simulink subsystem "Modulador_Tensiones"  (R2026a)
settings: Solver=VariableStepAuto
values from neighbouring files (symbols this model uses):
  L_d = 6.6e-3    (= 0.0066)    [coeficientes.m]
  L_q = 5.8e-3    (= 0.0058)    [coeficientes.m]
  lambda = 0.016    [coeficientes.m]
  Pp = 3    [coeficientes.m]
libraries: eeTransforms x2
settings Model: Creator=admin  LastModifiedBy=admin

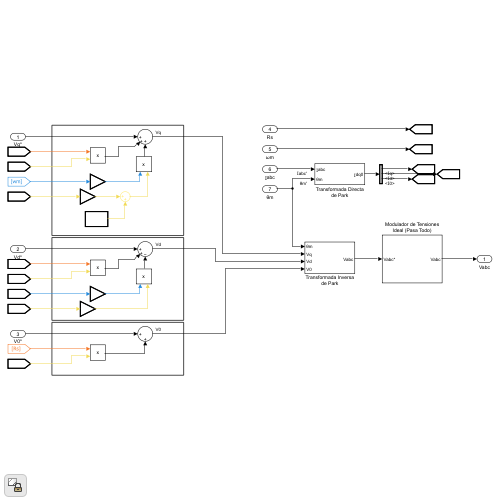
[thumbnail: Simulink's stored preview of the top-level diagram]
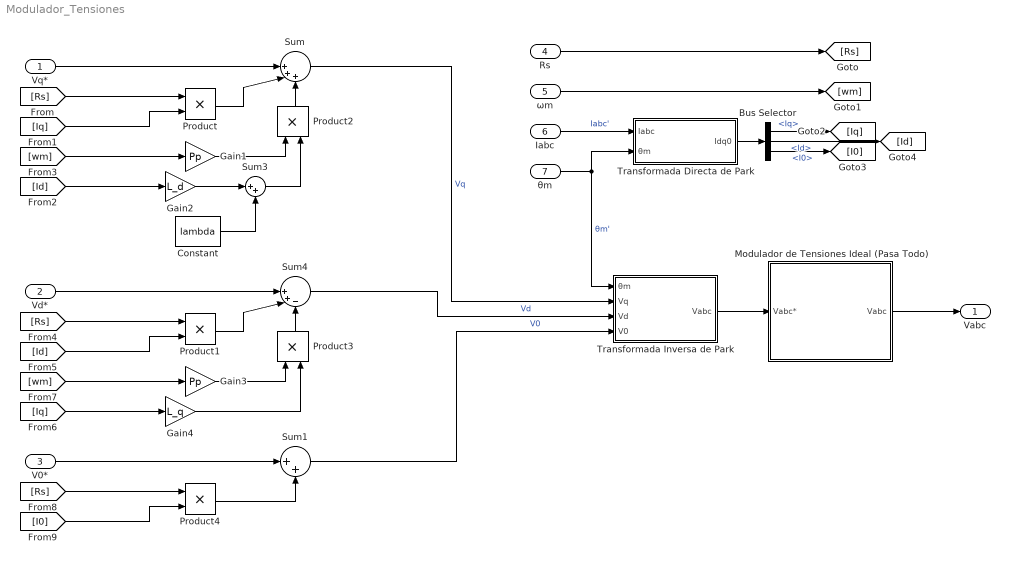
== system Modulador_Tensiones ==
  Vq* : Inport
  Vd* : Inport  Port=2
  V0* : Inport  Port=3
  Rs : Inport  Port=4
  ωm : Inport  Port=5
  Ⅰabc : Inport  Port=6
  θm : Inport  Port=7
  Bus Selector : BusSelector  OutputSignals=Ⅰq,Ⅰd,Ⅰ0
  Constant : Constant  Value=lambda
  Gain1 : Gain  Gain=Pp
  Gain2 : Gain  Gain=L_d
  Gain3 : Gain  Gain=Pp
  Gain4 : Gain  Gain=L_q
  Modulador de Tensiones Ideal (Pasa Todo) : Subsystem
  Product{,1..4} (5 alike) : Product
  Sum : Sum  Inputs=||+++
  Sum1 : Sum  Inputs=|++
  Sum3 : Sum  Inputs=|++
  Sum4 : Sum  Inputs=||++-
  Transformada Directa de Park : Subsystem
  Transformada Inversa de Park : Subsystem
  Vabc : Outport
  wires:
  Sum1/1 -> Transformada Inversa de Park/4(V0)  "V0"
  Sum4/1 -> Transformada Inversa de Park/3(Vd)  "Vd"
  Sum/1 -> Transformada Inversa de Park/2(Vq)  "Vq"
  Product4/1 -> Sum1/2
  V0*/1 -> Sum1/1
  [Rs] -> Product4/1
  [I0] -> Product4/2
  [Id] -> Product1/2
  Product3/1 -> Sum4/3
  Gain4/1 -> Product3/2
  Vd*/1 -> Sum4/1
  [Rs] -> Product1/1
  Gain3/1 -> Product3/1
  [Iq] -> Gain4/1
  Product1/1 -> Sum4/2
  [wm] -> Gain3/1
  [Iq] -> Product/2
  Gain1/1 -> Product2/1
  Sum3/1 -> Product2/2
  [wm] -> Gain1/1
  Product2/1 -> Sum/3
  Gain2/1 -> Sum3/1
  [Id] -> Gain2/1
  Constant/1 -> Sum3/2
  Product/1 -> Sum/2
  [Rs] -> Product/1
  Vq*/1 -> Sum/1
  Bus Selector/2 -> [Id]  "<Ⅰd>"
  Bus Selector/3 -> [I0]  "<Ⅰ0>"
  Bus Selector/1 -> [Iq]  "<Ⅰq>"
  ωm/1 -> [wm]
  Rs/1 -> [Rs]
  Transformada Inversa de Park/1(Vabc) -> Modulador de Tensiones Ideal (Pasa Todo)/1(Vabc*)
  Modulador de Tensiones Ideal (Pasa Todo)/1(Vabc) -> Vabc/1
  θm/1 -> Transformada Inversa de Park/1(θm), Transformada Directa de Park/2(θm)  "θm'"
  Transformada Directa de Park/1(Ⅰdq0) -> Bus Selector/1
  Ⅰabc/1 -> Transformada Directa de Park/1(Ⅰabc)  "Ⅰabc'"

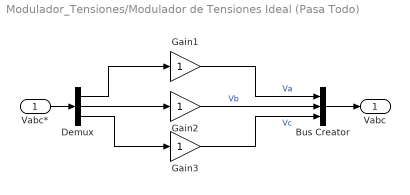
== system Modulador_Tensiones/Modulador de Tensiones Ideal (Pasa Todo) ==
  Vabc* : Inport
  Bus Creator : BusCreator  Inputs=3
  Demux : Demux  Outputs=3
  Gain1 : Gain
  Gain2 : Gain
  Gain3 : Gain
  Vabc : Outport
  wires:
  Bus Creator/1 -> Vabc/1
  Demux/3 -> Gain3/1
  Demux/1 -> Gain1/1
  Vabc*/1 -> Demux/1
  Demux/2 -> Gain2/1
  Gain1/1 -> Bus Creator/1  "Va"
  Gain3/1 -> Bus Creator/3  "Vc"
  Gain2/1 -> Bus Creator/2  "Vb"

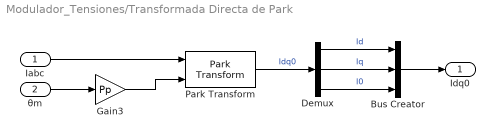
== system Modulador_Tensiones/Transformada Directa de Park ==
  Ⅰabc : Inport
  θm : Inport  Port=2
  Bus Creator : BusCreator  Inputs=3
  Demux : Demux  Outputs=3
  Gain3 : Gain  Gain=Pp
  Park Transform : eeTransforms/Park Transform  AxisAlignment=Q-axis  PowerInvariant=off
      settings: LibrarySourceBlock=|
      | ee_sl_lib/Mathematical
      | Transforms/Park Transform
  Ⅰdq0 : Outport
  wires:
  θm/1 -> Gain3/1
  Ⅰabc/1 -> Park Transform/1
  Bus Creator/1 -> Ⅰdq0/1
  Demux/2 -> Bus Creator/2  "Ⅰq"
  Demux/3 -> Bus Creator/3  "Ⅰ0"
  Demux/1 -> Bus Creator/1  "Ⅰd"
  Park Transform/1 -> Demux/1  "Ⅰdq0"
  Gain3/1 -> Park Transform/2

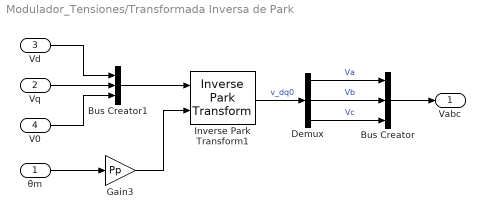
== system Modulador_Tensiones/Transformada Inversa de Park ==
  θm : Inport
  Vq : Inport  Port=2
  Vd : Inport  Port=3
  V0 : Inport  Port=4
  Bus Creator : BusCreator  Inputs=3
  Bus Creator1 : BusCreator  Inputs=3
  Demux : Demux  Outputs=3
  Gain3 : Gain  Gain=Pp
  Inverse Park Transform1 : eeTransforms/Inverse Park Transform  AxisAlignment=Q-axis  PowerInvariant=off
      settings: LibrarySourceBlock=|
      | ee_sl_lib/Mathematical
      | Transforms/Inverse
      | Park Transform
  Vabc : Outport
  wires:
  Bus Creator1/1 -> Inverse Park Transform1/1
  V0/1 -> Bus Creator1/3
  Vq/1 -> Bus Creator1/2
  Vd/1 -> Bus Creator1/1
  θm/1 -> Gain3/1
  Bus Creator/1 -> Vabc/1
  Demux/2 -> Bus Creator/2  "Vb"
  Demux/3 -> Bus Creator/3  "Vc"
  Demux/1 -> Bus Creator/1  "Va"
  Inverse Park Transform1/1 -> Demux/1  "v_dq0"
  Gain3/1 -> Inverse Park Transform1/2
